simulink model "v2_3_debug3"  (R2017a)
settings: Solver=VariableStepAuto  StartTime=0.0  StopTime=50  RelTol=1e-3
undefined symbols (not defined in the file): EbN0, TracebackDepth
libraries: commdigbbndpm3 x3, commcnvcod2 x2, commblkintrlv2 x2, commchan3 x2, commrandsrc3 x1, dspmtrx3 x1, commsink2 x1, dspstat3 x1, dspquant2 x1
settings Model: Creator=DELL  LastModifiedBy=DELL

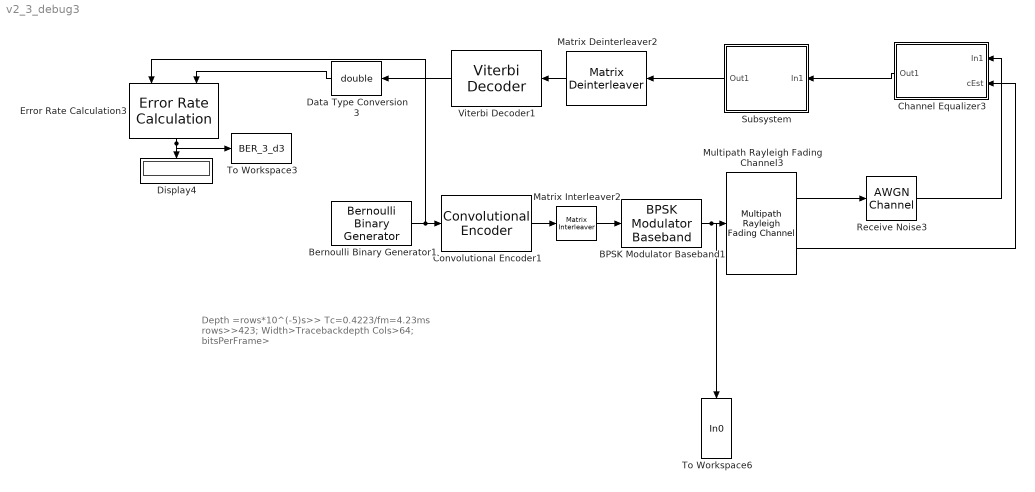
== system v2_3_debug3 ==
  note: Depth =rows*10^(-5)s>> Tc=0.4223/fm=4.23ms
      | 	rows>>423;
      |
      | Width>Tracebackdepth
      | 	Cols>64;
      |
      | bitsPerFrame>
  BPSK Modulator Baseband1 : commdigbbndpm3/BPSK Modulator Baseband  Ph=0  outDtype=double  outWordLen=16  outUDDataType=sfix(16)  outFracLenMode=Best precision  outFracLen=15  outDataTypeStr=double  outLastDataTypeStr=double
  Bernoulli Binary Generator1 : commrandsrc3/Bernoulli Binary Generator  ProbabilityOfZero=0.5  SeedSource=Auto  Seed=0  SampleTime=1e-5  SamplesPerFrame=SamplesPerFrame  OutputDataType=double  SimulateUsing=Interpreted execution
  Channel Equalizer3 : Subsystem
      mask Display:
      | disp('Equalizer');
      | port_label('input', 2, 'cEst');
  Convolutional Encoder1 : commcnvcod2/Convolutional Encoder  trellis=poly2trellis(9, [561 753])  opMode=Continuous  DelayedResetAction=off  hasIniStPort=off  hasFinStPort=off  usePuncVector=off  punctureVector=[1; 1; 0; 1; 0; 1]  reset=Unused parameter value
      settings: SourceProductName=Communications System Toolbox  SourceProductBaseCode=CM
  Data Type Conversion3 : DataTypeConversion  OutDataTypeStr=double
  Display4 : Display
  Error Rate Calculation3 : commsink2/Error Rate Calculation  N=TracebackDepth  st_delay=0  cp_mode=Entire frame  subframe=[]  PMode=Port  WsName=ErrorVec  RsMode2=off  stop=off  numErr=100  maxBits=1e6
  Matrix Deinterleaver2 : commblkintrlv2/Matrix Deinterleaver  Nrows=Rows  Ncols=Cols
      settings: SourceProductName=Communications System Toolbox  SourceProductBaseCode=CM
  Matrix Interleaver2 : commblkintrlv2/Matrix Interleaver  Nrows=Rows  Ncols=Cols
      settings: SourceProductName=Communications System Toolbox  SourceProductBaseCode=CM
  Multipath Rayleigh Fading Channel3 : commchan3/Multipath Rayleigh Fading Channel  maxDopplerShift=100  spectrumType=Jakes  sigmaGaussian=1/sqrt(2)  coeffRounded=[1 -1.72 0.785]  freqMinMaxRJakes=[0 1]  freqMinMaxAJakes=[0 1]  sigmaGaussian1=1/sqrt(2)  sigmaGaussian2=1/sqrt(2)  centerFreqGaussian1=0.0  centerFreqGaussian2=0.0  gainGaussian1=0.5  gainGaussian2=0.5  coeffBell=9  dopplerSpectrum=doppler.jakes  pathDelays=0  avgPathGaindB=2  normalizePathGains=on  seed=12345  enableProbe=0  openVisAtStart=off  outPathGains=on  outDelay=off
      settings: SourceProductName=Communications System Toolbox  SourceProductBaseCode=CM
  Receive Noise3 : commchan3/AWGN Channel  InputProcessing=Columns as channels (frame based)  seed=188  noiseMode="Signal to noise ratio  (Eb/No)"  EbNodB=EbN0  EsNodB=EbNo  SNRdB=50  bitsPerSym=1  Ps=1  Tsym=1e-5  variance=1
  Subsystem : Subsystem
      mask Display: disp('Soft-Output\nBPSK\nDemodulator')
  To Workspace3 : ToWorkspace  VariableName=BER_3_d3  SampleTime=-1
      settings: MaxDataPoints=1
  To Workspace6 : ToWorkspace  VariableName=In0  SampleTime=-1
      settings: MaxDataPoints=1
  Viterbi Decoder1 : commcnvcod2/Viterbi Decoder  trellis=poly2trellis(9, [561 753])  isPunctured=off  punctureVector=[1; 1; 0; 1; 0; 1]  erasures=off  dectype=Soft decision  nsdecb=8  runSigValErrCheck=off  tbdepth=TracebackDepth  opmode=Continuous  reset=off  delayedResetAction=off  smWordLength=16  outDataType=Inherit via internal rule
      settings: SourceProductName=Communications System Toolbox  SourceProductBaseCode=CM
  wires:
  BPSK Modulator Baseband1/1 -> To Workspace6/1, Multipath Rayleigh Fading Channel3/1
  Error Rate Calculation3/1 -> To Workspace3/1, Display4/1
  Multipath Rayleigh Fading Channel3/2 -> Channel Equalizer3/2(cEst)
  Multipath Rayleigh Fading Channel3/1 -> Receive Noise3/1
  Channel Equalizer3/1(Out1) -> Subsystem/1(In1)
  Receive Noise3/1 -> Channel Equalizer3/1(In1)
  Data Type Conversion3/1 -> Error Rate Calculation3/2
  Bernoulli Binary Generator1/1 -> Error Rate Calculation3/1, Convolutional Encoder1/1
  Matrix Interleaver2/1 -> BPSK Modulator Baseband1/1
  Matrix Deinterleaver2/1 -> Viterbi Decoder1/1
  Convolutional Encoder1/1 -> Matrix Interleaver2/1
  Viterbi Decoder1/1 -> Data Type Conversion3/1
  Subsystem/1(Out1) -> Matrix Deinterleaver2/1

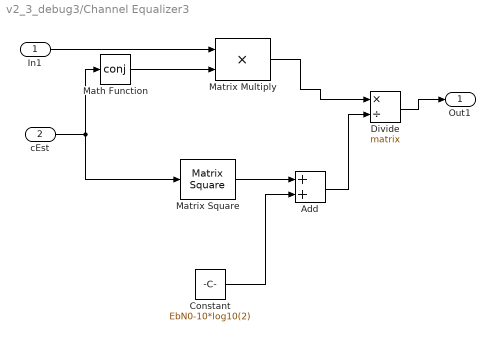
== system v2_3_debug3/Channel Equalizer3 ==
  In1 : Inport
  cEst : Inport  Port=2
  Add : Sum
  Constant : Constant  Value=EbN0-10*log10(2)
  Divide : Product  Inputs=*/  Multiplication=Matrix(*)
  Math Function : Math  Operator=conj  SaturateOnIntegerOverflow=on
  Matrix Square : dspmtrx3/Matrix Square  OutMin=[]  OutMax=[]
      settings: SourceProductName=DSP System Toolbox  SourceProductBaseCode=DS
  Matrix Multiply : Product
  Out1 : Outport
  wires:
  In1/1 -> Matrix Multiply/1
  cEst/1 -> Matrix Square/1, Math Function/1
  Matrix Multiply/1 -> Divide/1
  Divide/1 -> Out1/1
  Math Function/1 -> Matrix Multiply/2
  Matrix Square/1 -> Add/1
  Add/1 -> Divide/2
  Constant/1 -> Add/2

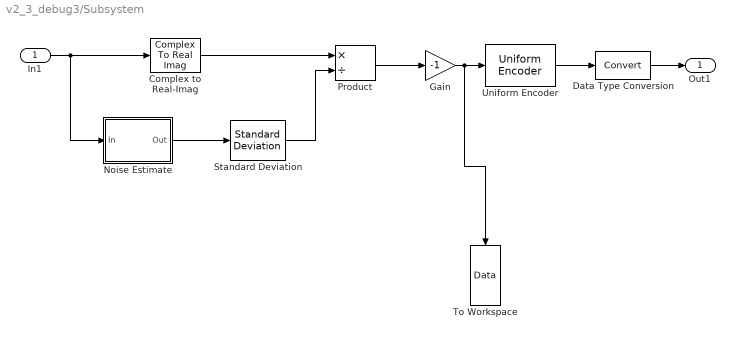
== system v2_3_debug3/Subsystem ==
  In1 : Inport
  Complex to Real-Imag : ComplexToRealImag  Output=Real
  Data Type Conversion : DataTypeConversion  SaturateOnIntegerOverflow=on  RndMeth=Zero
  Gain : Gain  Gain=-1  SaturateOnIntegerOverflow=on  OutDataTypeStr=Inherit: Same as input  ParamDataTypeStr=Inherit: Same as input
  Noise Estimate : Subsystem
  Product : Product  Inputs=*/  SaturateOnIntegerOverflow=on  RndMeth=Zero  InputSameDT=on  OutDataTypeStr=Inherit: Same as first input
  Standard Deviation : dspstat3/Standard Deviation  run=off  directionMode=Each column  dimension=1  InputProcessing=Columns as channels (frame based)  reset_popup=None  roiEnable=off  roiType=Rectangles  roiPortion=Entire ROI  roiOutput=Individual statistics for each ROI  roiFlag=off
      settings: SourceProductName=DSP System Toolbox  SourceProductBaseCode=DS
  To Workspace : ToWorkspace  VariableName=Data  SampleTime=-1
      settings: MaxDataPoints=1
  Uniform Encoder : dspquant2/Uniform Encoder  peak=0.001  bits=8  otype=Unsigned integer
      settings: SourceProductName=DSP System Toolbox
  Out1 : Outport
  wires:
  Standard Deviation/1 -> Product/2
  In1/1 -> Complex to Real-Imag/1, Noise Estimate/1(In)
  Complex to Real-Imag/1 -> Product/1
  Uniform Encoder/1 -> Data Type Conversion/1
  Gain/1 -> To Workspace/1, Uniform Encoder/1
  Product/1 -> Gain/1
  Data Type Conversion/1 -> Out1/1
  Noise Estimate/1(Out) -> Standard Deviation/1

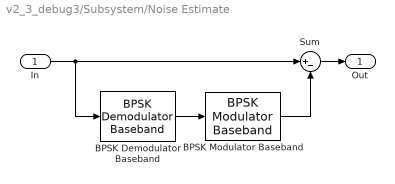
== system v2_3_debug3/Subsystem/Noise Estimate ==
  In : Inport
  BPSK Demodulator Baseband : commdigbbndpm3/BPSK Demodulator Baseband  DecType=Hard decision  VarSource=Dialog  Variance=1  Ph=0  outDtype=Inherit via internal rule  derotateFactorWordLen=16  derotateFactorDataTypeStr=Inherit: Same word length as input  derotateFactorLastDataTypeStr=Inherit: Same word length as input
  BPSK Modulator Baseband : commdigbbndpm3/BPSK Modulator Baseband  Ph=0  outDtype=double  outWordLen=16  outUDDataType=sfix(16)  outFracLenMode=Best precision  outFracLen=15  outDataTypeStr=double  outLastDataTypeStr=double
  Sum : Sum  Inputs=|+-  SaturateOnIntegerOverflow=on
  Out : Outport
  wires:
  Sum/1 -> Out/1
  In/1 -> Sum/1, BPSK Demodulator Baseband/1
  BPSK Modulator Baseband/1 -> Sum/2
  BPSK Demodulator Baseband/1 -> BPSK Modulator Baseband/1
